simulink model "theta_cmd"  (R2019a)
settings: Solver=VariableStepAuto  StartTime=0.0  StopTime=200  RelTol=1e-3
values from neighbouring files (symbols this model uses):
  A1 = [X_u+X_T_u X_alpha 0 -g*cos(theta_1) ... (first row only)    [Rocket_Control_NeuroFuzzy.m]    (also in Space_Stade.m)
  B1 = [X_de ... (first row only)    [Rocket_Control_NeuroFuzzy.m]    (also in Space_Stade.m)
  C1 = [1 0 0 0 ... (first row only)    [Rocket_Control_NeuroFuzzy.m]    (also in Space_Stade.m)
  D1 = [0 ... (first row only)    [Rocket_Control_NeuroFuzzy.m]    (also in Space_Stade.m)
  U_1 = 0.35*340    (= 119)    [Rocket_Control_NeuroFuzzy.m]    (also in Space_Stade.m)
libraries: simulink x1
settings Model: Creator=yuril  LastModifiedBy=yuril

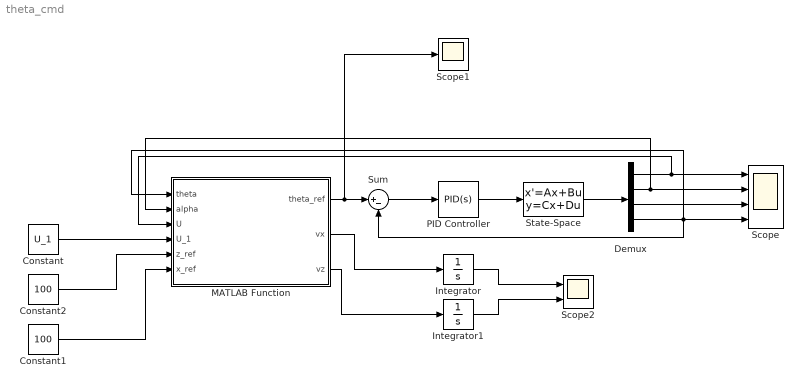
== system theta_cmd ==
  Constant : Constant  Value=U_1
  Constant1 : Constant  Value=100
  Constant2 : Constant  Value=100
  Demux : Demux
  Integrator : Integrator
  Integrator1 : Integrator
  MATLAB Function : MATLAB Function  TreatAsAtomicUnit=on
  PID Controller : simulink/Continuous/PID Controller  Controller=PID  Form=Parallel  TimeDomain=Continuous-time  SampleTime=-1  IntegratorMethod=Forward Euler  FilterMethod=Forward Euler  ControllerParametersSource=internal  P=-15.2840271392028  I=-2.0147445350613  D=43.8056913675579  UseFilter=on  N=0.348905054618589  TunerSelectOption=Transfer Function Based (PID Tuner App)  InitialConditionSource=internal  InitialConditionForIntegrator=0  InitialConditionForFilter=0  DifferentiatorICPrevScaledInput=0  ExternalReset=none  TrackingMode=off  Kt=1  LimitOutput=off  UpperSaturationLimit=inf  LowerSaturationLimit=-inf  LinearizeAsGain=on  AntiWindupMode=none  Kb=1  POutMin=[]  POutMax=[]  IOutMin=[]  IOutMax=[]  DOutMin=[]  DOutMax=[]  NOutMin=[]  NOutMax=[]  SumOutMin=[]  SumOutMax=[]  SaturationOutMin=[]  SaturationOutMax=[]  PParamMin=[]  PParamMax=[]  IParamMin=[]  IParamMax=[]  DParamMin=[]  DParamMax=[]  NParamMin=[]  NParamMax=[]  KbParamMin=[]  KbParamMax=[]  KtParamMin=[]  KtParamMax=[]  KbOutMin=[]  KbOutMax=[]  KtOutMin=[]  KtOutMax=[]  IntegratorOutMin=[]  IntegratorOutMax=[]  FilterOutMin=[]  FilterOutMax=[]  SumI1OutMin=[]  SumI1OutMax=[]  SumI2OutMin=[]  SumI2OutMax=[]  SumI3OutMin=[]  SumI3OutMax=[]  SumI4OutMin=[]  SumI4OutMax=[]  SumDOutMin=[]  SumDOutMax=[]  DifferentiatorOutMin=[]  DifferentiatorOutMax=[]  FilterDiffOutCoefMin=[]  FilterDiffOutCoefMax=[]  ReciprocalOutMin=[]  ReciprocalOutMax=[]  SumDenOutMin=[]  SumDenOutMax=[]  SumNumOutMin=[]  SumNumOutMax=[]  DivideOutMin=[]  DivideOutMax=[]  IntegratorContinuousStateAttributes=''  IntegratorStateMustResolveToSignalObject=off  IntegratorRTWStateStorageClass=Auto  FilterContinuousStateAttributes=''  FilterStateMustResolveToSignalObject=off  FilterRTWStateStorageClass=Auto  ParallelPVariant=InternalParameters  IdealPVariant=Disabled  IVariant=InternalParameters  DVariant=InternalParameters  IntegratorVariant=Continuous  SatVariant=Disabled  AWVariant=Passthrough  PCopyVariant=Disabled  TRVariant=Disabled  FdbkBlocksVariant=Forward  IdealPFdbkVariant=Disabled  SatFdbkVariant=Disabled  DerivativeFilterVariant=ContFilter  NVariant=InternalParameters  NCopyVariant=Disabled  FilterICVariant=InternalICsFilter  IntegratorICVariant=InternalICs  ExternalResetVariant=Disabled  TRSumVariant=Passthrough  SumFdbkVariant=Disabled  SumVariant=Sum_PID
  Scope : Scope  NumInputPorts=4
  Scope1 : Scope
  Scope2 : Scope  NumInputPorts=2
  State-Space : StateSpace  A=A1  B=B1  C=C1  D=D1  InitialCondition=0
  Sum : Sum  Inputs=|+-
  wires:
  Constant/1 -> MATLAB Function/4(U_1)
  Constant2/1 -> MATLAB Function/5(z_ref)
  Constant1/1 -> MATLAB Function/6(x_ref)
  PID Controller/1 -> State-Space/1
  State-Space/1 -> Demux/1
  Demux/1 -> Scope/1, MATLAB Function/3(U)
  Demux/2 -> Scope/2, MATLAB Function/2(alpha)
  Sum/1 -> PID Controller/1
  MATLAB Function/1(theta_ref) -> Sum/1, Scope1/1
  Demux/4 -> Scope/4, MATLAB Function/1(theta), Sum/2
  Demux/3 -> Scope/3
  MATLAB Function/2(vx) -> Integrator/1
  MATLAB Function/3(vz) -> Integrator1/1
  Integrator/1 -> Scope2/1
  Integrator1/1 -> Scope2/2

== matlab function theta_cmd/MATLAB Function ==
  data: theta input; theta_ref output; alpha input; U input; U_1 input; z_ref input; x_ref input; vx output; vz output
function [theta_ref, vx, vz] = theta_cmd(theta, alpha, U, U_1, z_ref, x_ref)

vx = cos(theta)*U - sin(theta)*alpha*U_1;
vz = sin(theta)*U + cos(theta)*alpha*U_1;
% if vx == 0
%     vx = 1;
%     vz = 0;
% end
% gamma = atan(vz/vx);
% gamma_ref = atan(z_ref/x_ref);
% gamma_des = gamma_ref - gamma;
gamma_des = atan(0.3);
theta_ref = gamma_des + alpha;
end
